simulink subsystem "LEDs2"  (R2024b)
settings: Solver=VariableStepAuto  StartTime=0.0  StopTime=10.0  RelTol=1e-3
libraries: arduinolib x3, simulink x1
settings Model: Creator=Laura  LastModifiedBy=Laura

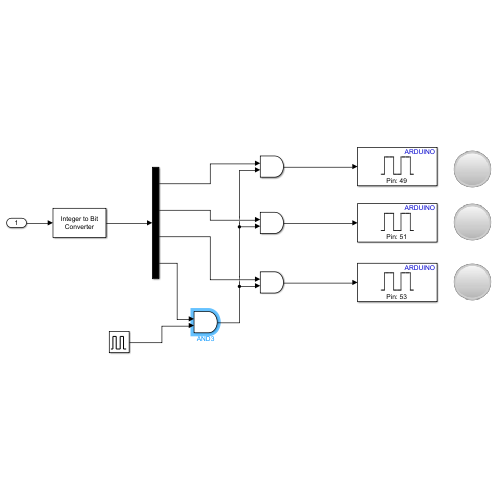
[thumbnail: Simulink's stored preview of the top-level diagram]
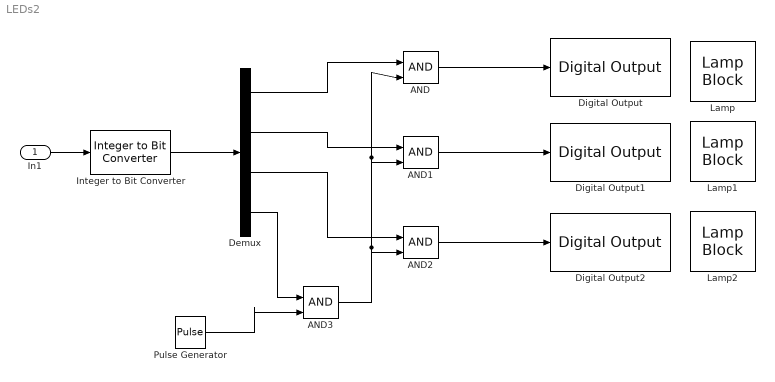
== system LEDs2 ==
  In1 : Inport
  AND{,1..3} (4 alike) : Logic  IconShape=distinctive  AllPortsSameDT=off  OutDataTypeStr=boolean
  Demux : Demux
  Digital Output : arduinolib/Digital Output  pinNumber=49  Direction=output  blockPlatform=arduino
  Digital Output1 : arduinolib/Digital Output  pinNumber=51  Direction=output  blockPlatform=arduino
  Digital Output2 : arduinolib/Digital Output  pinNumber=53  Direction=output  blockPlatform=arduino
  Integer to Bit Converter : simulink/Logic and Bit Operations/Integer to Bit Converter  nbits=4  signedInputValues=Unsigned  bitOrder=MSB first  outDtype=Inherit via internal rule
  Lamp : LampBlock  LabelPosition=Hide
  Lamp1 : LampBlock  LabelPosition=Hide
  Lamp2 : LampBlock  LabelPosition=Hide
  Pulse Generator : DiscretePulseGenerator  PulseType=Time based  Period=10  PulseWidth=5
  wires:
  Integer to Bit Converter/1 -> Demux/1
  In1/1 -> Integer to Bit Converter/1
  Demux/1 -> AND/1
  AND/1 -> Digital Output/1
  AND1/1 -> Digital Output1/1
  AND2/1 -> Digital Output2/1
  Demux/2 -> AND1/1
  Demux/3 -> AND2/1
  AND3/1 -> AND2/2, AND1/2, AND/2
  Demux/4 -> AND3/1
  Pulse Generator/1 -> AND3/2
